simulink model "cost_function_only"  (R2022a)
settings: Solver=FixedStepDiscrete  StartTime=0.0  StopTime=10.0  RelTol=1e-3
undefined symbols (not defined in the file or in its folder): f_c
libraries: hdlsllib x1
settings Model: DataTypeOverride=Off  Creator=Andre Merx  LastModifiedBy=Andre Merx
settings SolverCC: AlgebraicLoopSolver=TrustRegion
settings DataIOCC: LimitDataPoints=on  SaveOutput=off  SaveTime=off
settings OptimizationCC: BlockReduction=off  ConditionallyExecuteInputs=off  DefaultParameterBehavior=Inlined  LifeSpan=inf
settings DebuggingCC: AlgebraicLoopMsg=error  SingleTaskRateTransMsg=error  UnconnectedInputMsg=warning  UnconnectedOutputMsg=warning  UnconnectedLineMsg=warning  AllowSymbolicDim=off  StrictBusMsg=ErrorOnBusTreatedAsVector  SFUnexpectedBacktrackingDiag=warning  SFNoUnconditionalDefaultTransitionDiag=warning  SFExecutionAtInitializationDiag=none  SFMachineParentedDataDiag=warning  ArithmeticOperatorsInVariantConditions=warning
settings HardwareCC: ProdBitPerPointer=32  ProdBitPerSizeT=32  ProdBitPerPtrDiffT=32  ProdLargestAtomicFloat=None  ProdIntDivRoundTo=Undefined  ProdEndianess=Unspecified  ProdWordSize=32  ProdHWDeviceType=ASIC/FPGA->ASIC/FPGA  ProdEqTarget=off
settings SFSimCC: SimUseLocalCustomCode=off  CustomCodeUndefinedFunction=UseInterfaceOnly
settings RTWCC: RTWUseLocalCustomCode=off
settings CodeAppCC: StateflowObjectComments=on
settings GRTTargetCC: TargetLangStandard=C89/C90 (ANSI)
settings ConfigComp: CovScope=ReferencedModels  CovMetricSettings=dw  CovSaveCumulativeToWorkspaceVar=on  CovSaveSingleToWorkspaceVar=on  CovExternalEMLEnable=off  CovSFcnEnable=off

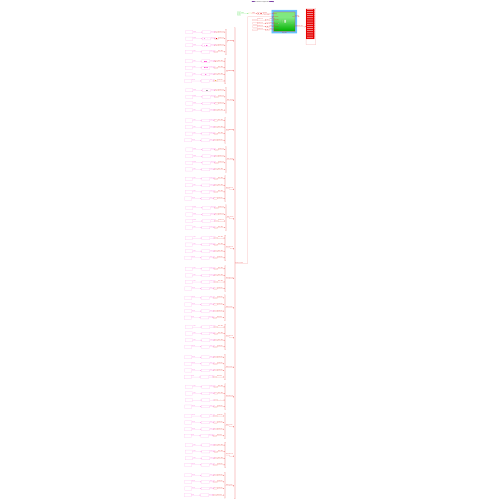
[thumbnail: Simulink's stored preview of the top-level diagram]
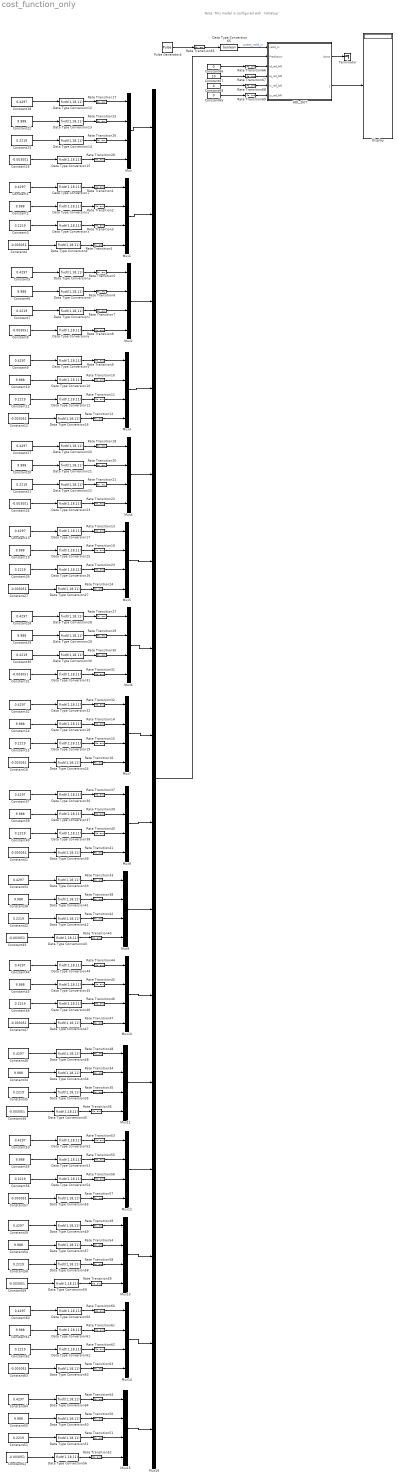
== system cost_function_only ==
  note: Note: This model is configured with ' hdlsetup '
  Constant{1,5,9,13,17..18,28,32..33,37,44,48..49,53,60,64} (16 alike) : Constant  Value=0.4297
  Constant{2,6,10,14,19..20,22,29,34,38..39,45,50,54..55,61} (16 alike) : Constant  Value=9.988
  Constant{3,7,11,15,21,23,26,30,35,40,42,46,51,56,58,62} (16 alike) : Constant  Value=0.2219
  Constant{4,8,12,16,24..25,27,31,36,41,43,47,52,57,59,63} (16 alike) : Constant  Value=-0.003051
  Constant65 : Constant  Value=0  OutDataTypeStr=fixdt(1,18,11)  SampleTime=-1
  Constant66 : Constant  Value=0  OutDataTypeStr=fixdt(1,18,11)  SampleTime=-1
  Constant67 : Constant  Value=10  OutDataTypeStr=fixdt(1,18,11)  SampleTime=-1
  Constant68 : Constant  Value=0  OutDataTypeStr=fixdt(1,18,11)  SampleTime=-1
  Data Type Conversion{1..64} (64 alike) : DataTypeConversion  OutDataTypeStr=fixdt(1,18,11)  SaturateOnIntegerOverflow=off  RndMeth=Floor
  Data Type Conversion65 : DataTypeConversion  OutDataTypeStr=boolean  SaturateOnIntegerOverflow=off  RndMeth=Floor
  Display : Display
  HDL_DUT : Subsystem  TreatAsAtomicUnit=on
  Mux{,1..15} (16 alike) : Mux
  Mux16 : Mux  Inputs=16
  Pulse Generator4 : DiscretePulseGenerator  PulseType=Time based  Period=1/f_c
  Rate Transition{1..69} (69 alike) : RateTransition  OutPortSampleTime=Rt
  Terminator : Terminator
  wires:
  Rate Transition17/1 -> Mux/1
  Constant25/1 -> Data Type Conversion15/1
  Rate Transition26/1 -> Mux/3
  Data Type Conversion12/1 -> Rate Transition17/1
  Rate Transition28/1 -> Mux/4
  Data Type Conversion13/1 -> Rate Transition25/1
  Data Type Conversion15/1 -> Rate Transition28/1
  Rate Transition25/1 -> Mux/2
  Constant18/1 -> Data Type Conversion12/1
  Constant23/1 -> Data Type Conversion14/1
  Constant22/1 -> Data Type Conversion13/1
  Data Type Conversion14/1 -> Rate Transition26/1
  Rate Transition4/1 -> Mux1/4
  Rate Transition3/1 -> Mux1/3
  Rate Transition2/1 -> Mux1/2
  Rate Transition1/1 -> Mux1/1
  Constant2/1 -> Data Type Conversion2/1
  Constant1/1 -> Data Type Conversion1/1
  Data Type Conversion4/1 -> Rate Transition4/1
  Constant3/1 -> Data Type Conversion3/1
  Data Type Conversion2/1 -> Rate Transition2/1
  Data Type Conversion1/1 -> Rate Transition1/1
  Constant4/1 -> Data Type Conversion4/1
  Data Type Conversion3/1 -> Rate Transition3/1
  Rate Transition8/1 -> Mux2/4
  Rate Transition7/1 -> Mux2/3
  Rate Transition6/1 -> Mux2/2
  Rate Transition5/1 -> Mux2/1
  Constant6/1 -> Data Type Conversion6/1
  Constant5/1 -> Data Type Conversion5/1
  Data Type Conversion8/1 -> Rate Transition8/1
  Constant7/1 -> Data Type Conversion7/1
  Data Type Conversion6/1 -> Rate Transition6/1
  Data Type Conversion5/1 -> Rate Transition5/1
  Constant8/1 -> Data Type Conversion8/1
  Data Type Conversion7/1 -> Rate Transition7/1
  Rate Transition12/1 -> Mux3/4
  Rate Transition11/1 -> Mux3/3
  Rate Transition10/1 -> Mux3/2
  Rate Transition9/1 -> Mux3/1
  Constant10/1 -> Data Type Conversion10/1
  Constant9/1 -> Data Type Conversion9/1
  Data Type Conversion16/1 -> Rate Transition12/1
  Constant11/1 -> Data Type Conversion11/1
  Data Type Conversion10/1 -> Rate Transition10/1
  Data Type Conversion9/1 -> Rate Transition9/1
  Constant12/1 -> Data Type Conversion16/1
  Data Type Conversion11/1 -> Rate Transition11/1
  Rate Transition22/1 -> Mux4/4
  Rate Transition21/1 -> Mux4/3
  Rate Transition20/1 -> Mux4/2
  Data Type Conversion20/1 -> Rate Transition18/1
  Constant17/1 -> Data Type Conversion20/1
  Constant21/1 -> Data Type Conversion22/1
  Data Type Conversion21/1 -> Rate Transition20/1
  Data Type Conversion22/1 -> Rate Transition21/1
  Data Type Conversion30/1 -> Rate Transition30/1
  Constant31/1 -> Data Type Conversion31/1
  Constant24/1 -> Data Type Conversion23/1
  Data Type Conversion28/1 -> Rate Transition27/1
  Data Type Conversion29/1 -> Rate Transition29/1
  Constant30/1 -> Data Type Conversion30/1
  Constant20/1 -> Data Type Conversion21/1
  Constant28/1 -> Data Type Conversion28/1
  Data Type Conversion31/1 -> Rate Transition31/1
  Rate Transition27/1 -> Mux6/1
  Rate Transition29/1 -> Mux6/2
  Rate Transition30/1 -> Mux6/3
  Rate Transition31/1 -> Mux6/4
  Rate Transition24/1 -> Mux5/4
  Data Type Conversion17/1 -> Rate Transition13/1
  Data Type Conversion25/1 -> Rate Transition19/1
  Constant19/1 -> Data Type Conversion25/1
  Rate Transition13/1 -> Mux5/1
  Constant26/1 -> Data Type Conversion26/1
  Rate Transition19/1 -> Mux5/2
  Rate Transition23/1 -> Mux5/3
  Rate Transition18/1 -> Mux4/1
  Constant16/1 -> Data Type Conversion24/1
  Data Type Conversion19/1 -> Rate Transition15/1
  Data Type Conversion23/1 -> Rate Transition22/1
  Data Type Conversion18/1 -> Rate Transition14/1
  Data Type Conversion26/1 -> Rate Transition23/1
  Data Type Conversion32/1 -> Rate Transition32/1
  Constant13/1 -> Data Type Conversion17/1
  Data Type Conversion24/1 -> Rate Transition16/1
  Constant32/1 -> Data Type Conversion32/1
  Constant14/1 -> Data Type Conversion18/1
  Constant15/1 -> Data Type Conversion19/1
  Constant29/1 -> Data Type Conversion29/1
  Rate Transition15/1 -> Mux7/3
  Constant27/1 -> Data Type Conversion27/1
  Rate Transition14/1 -> Mux7/2
  Rate Transition16/1 -> Mux7/4
  Data Type Conversion27/1 -> Rate Transition24/1
  Rate Transition32/1 -> Mux7/1
  Rate Transition41/1 -> Mux8/4
  Rate Transition40/1 -> Mux8/3
  Rate Transition39/1 -> Mux8/2
  Data Type Conversion36/1 -> Rate Transition37/1
  Constant37/1 -> Data Type Conversion36/1
  Constant40/1 -> Data Type Conversion38/1
  Data Type Conversion37/1 -> Rate Transition39/1
  Data Type Conversion38/1 -> Rate Transition40/1
  Data Type Conversion46/1 -> Rate Transition46/1
  Constant47/1 -> Data Type Conversion47/1
  Constant41/1 -> Data Type Conversion39/1
  Data Type Conversion44/1 -> Rate Transition44/1
  Data Type Conversion45/1 -> Rate Transition45/1
  Constant46/1 -> Data Type Conversion46/1
  Constant39/1 -> Data Type Conversion37/1
  Constant44/1 -> Data Type Conversion44/1
  Data Type Conversion47/1 -> Rate Transition47/1
  Rate Transition44/1 -> Mux10/1
  Rate Transition45/1 -> Mux10/2
  Rate Transition46/1 -> Mux10/3
  Rate Transition47/1 -> Mux10/4
  Rate Transition43/1 -> Mux9/4
  Data Type Conversion33/1 -> Rate Transition33/1
  Data Type Conversion41/1 -> Rate Transition38/1
  Constant38/1 -> Data Type Conversion41/1
  Rate Transition33/1 -> Mux9/1
  Constant42/1 -> Data Type Conversion42/1
  Rate Transition38/1 -> Mux9/2
  Rate Transition42/1 -> Mux9/3
  Rate Transition37/1 -> Mux8/1
  Constant36/1 -> Data Type Conversion40/1
  Data Type Conversion35/1 -> Rate Transition35/1
  Data Type Conversion39/1 -> Rate Transition41/1
  Data Type Conversion34/1 -> Rate Transition34/1
  Data Type Conversion42/1 -> Rate Transition42/1
  Data Type Conversion48/1 -> Rate Transition48/1
  Constant33/1 -> Data Type Conversion33/1
  Data Type Conversion40/1 -> Rate Transition36/1
  Constant48/1 -> Data Type Conversion48/1
  Constant34/1 -> Data Type Conversion34/1
  Constant35/1 -> Data Type Conversion35/1
  Constant45/1 -> Data Type Conversion45/1
  Rate Transition35/1 -> Mux11/3
  Constant43/1 -> Data Type Conversion43/1
  Rate Transition34/1 -> Mux11/2
  Rate Transition36/1 -> Mux11/4
  Data Type Conversion43/1 -> Rate Transition43/1
  Rate Transition48/1 -> Mux11/1
  Rate Transition57/1 -> Mux12/4
  Rate Transition56/1 -> Mux12/3
  Rate Transition55/1 -> Mux12/2
  Data Type Conversion52/1 -> Rate Transition53/1
  Constant53/1 -> Data Type Conversion52/1
  Constant56/1 -> Data Type Conversion54/1
  Data Type Conversion53/1 -> Rate Transition55/1
  Data Type Conversion54/1 -> Rate Transition56/1
  Data Type Conversion62/1 -> Rate Transition62/1
  Constant63/1 -> Data Type Conversion63/1
  Constant57/1 -> Data Type Conversion55/1
  Data Type Conversion60/1 -> Rate Transition60/1
  Data Type Conversion61/1 -> Rate Transition61/1
  Constant62/1 -> Data Type Conversion62/1
  Constant55/1 -> Data Type Conversion53/1
  Constant60/1 -> Data Type Conversion60/1
  Data Type Conversion63/1 -> Rate Transition63/1
  Rate Transition60/1 -> Mux14/1
  Rate Transition61/1 -> Mux14/2
  Rate Transition62/1 -> Mux14/3
  Rate Transition63/1 -> Mux14/4
  Rate Transition59/1 -> Mux13/4
  Data Type Conversion49/1 -> Rate Transition49/1
  Data Type Conversion57/1 -> Rate Transition54/1
  Constant54/1 -> Data Type Conversion57/1
  Rate Transition49/1 -> Mux13/1
  Constant58/1 -> Data Type Conversion58/1
  Rate Transition54/1 -> Mux13/2
  Rate Transition58/1 -> Mux13/3
  Rate Transition53/1 -> Mux12/1
  Constant52/1 -> Data Type Conversion56/1
  Data Type Conversion51/1 -> Rate Transition51/1
  Data Type Conversion55/1 -> Rate Transition57/1
  Data Type Conversion50/1 -> Rate Transition50/1
  Data Type Conversion58/1 -> Rate Transition58/1
  Data Type Conversion64/1 -> Rate Transition64/1
  Constant49/1 -> Data Type Conversion49/1
  Data Type Conversion56/1 -> Rate Transition52/1
  Constant64/1 -> Data Type Conversion64/1
  Constant50/1 -> Data Type Conversion50/1
  Constant51/1 -> Data Type Conversion51/1
  Constant61/1 -> Data Type Conversion61/1
  Rate Transition51/1 -> Mux15/3
  Constant59/1 -> Data Type Conversion59/1
  Rate Transition50/1 -> Mux15/2
  Rate Transition52/1 -> Mux15/4
  Data Type Conversion59/1 -> Rate Transition59/1
  Rate Transition64/1 -> Mux15/1
  Mux/1 -> Mux16/1
  Mux1/1 -> Mux16/2
  Mux2/1 -> Mux16/3
  Mux3/1 -> Mux16/4
  Mux4/1 -> Mux16/5
  Mux5/1 -> Mux16/6
  Mux6/1 -> Mux16/7
  Mux7/1 -> Mux16/8
  Mux8/1 -> Mux16/9
  Mux9/1 -> Mux16/10
  Mux10/1 -> Mux16/11
  Mux11/1 -> Mux16/12
  Mux12/1 -> Mux16/13
  Mux13/1 -> Mux16/14
  Mux14/1 -> Mux16/15
  Mux15/1 -> Mux16/16
  Mux16/1 -> HDL_DUT/2(Prediction)
  Data Type Conversion65/1 -> HDL_DUT/1(valid_in)  "curent_valid_in"
  Pulse Generator4/1 -> Rate Transition65/1
  Rate Transition65/1 -> Data Type Conversion65/1
  Constant67/1 -> Rate Transition67/1
  Constant66/1 -> Rate Transition66/1
  Rate Transition66/1 -> HDL_DUT/3(id_ref_AXI)
  Constant68/1 -> Rate Transition68/1
  Rate Transition68/1 -> HDL_DUT/5(ix_ref_AXI)
  Rate Transition67/1 -> HDL_DUT/4(iq_ref_AXI)
  Rate Transition69/1 -> HDL_DUT/6(iy_ref_AXI)
  Constant65/1 -> Rate Transition69/1
  HDL_DUT/1(done) -> Terminator/1
  HDL_DUT/2(J) -> Display/1

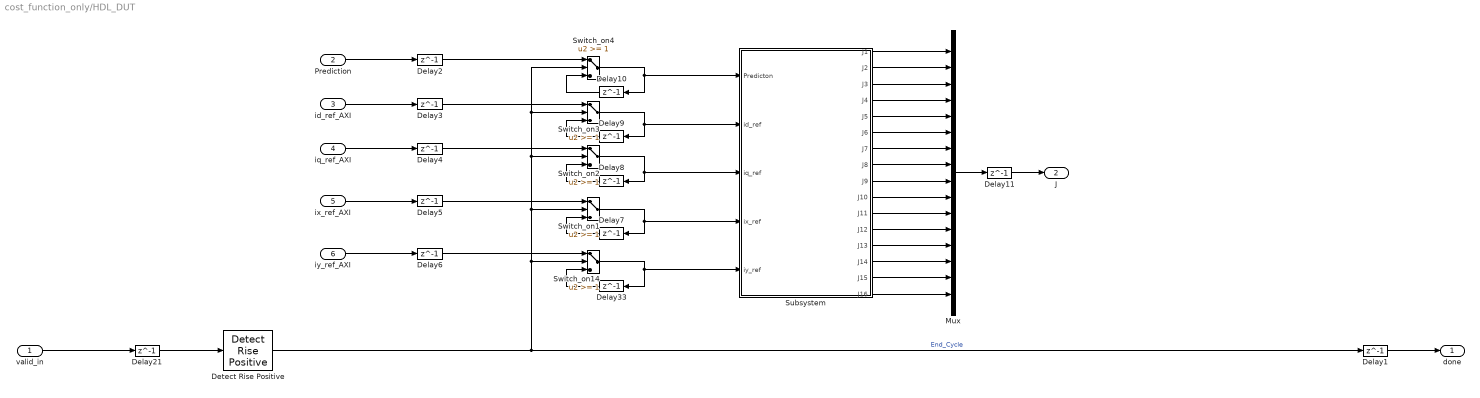
== system cost_function_only/HDL_DUT ==
  valid_in : Inport
  Prediction : Inport  Port=2
  id_ref_AXI : Inport  Port=3
  iq_ref_AXI : Inport  Port=4
  ix_ref_AXI : Inport  Port=5
  iy_ref_AXI : Inport  Port=6
  Delay{1..11,21,33} (13 alike) : Delay  DelayLength=1
  Detect Rise Positive : hdlsllib/Logic and Bit Operations/Detect Rise Positive  vinit=0  OutDataTypeStr=boolean
      settings: SourceProductBaseCode=SL
  Mux : Mux  Inputs=16
  Subsystem : Subsystem
  Switch_on{1..4,14} (5 alike) : Switch  Threshold=1  OutDataTypeStr=fixdt(1,18,11)  RndMeth=Simplest  SaturateOnIntegerOverflow=off  InputSameDT=off
  done : Outport
  J : Outport  Port=2
  wires:
  Delay21/1 -> Detect Rise Positive/1
  valid_in/1 -> Delay21/1
  Delay1/1 -> done/1
  Prediction/1 -> Delay2/1
  id_ref_AXI/1 -> Delay3/1
  iq_ref_AXI/1 -> Delay4/1
  ix_ref_AXI/1 -> Delay5/1
  iy_ref_AXI/1 -> Delay6/1
  Delay6/1 -> Switch_on14/1
  Switch_on14/1 -> Delay33/1, Subsystem/5(iy_ref)
  Delay33/1 -> Switch_on14/3
  Delay7/1 -> Switch_on1/3
  Delay5/1 -> Switch_on1/1
  Switch_on1/1 -> Subsystem/4(ix_ref), Delay7/1
  Delay8/1 -> Switch_on2/3
  Delay4/1 -> Switch_on2/1
  Switch_on2/1 -> Subsystem/3(iq_ref), Delay8/1
  Delay9/1 -> Switch_on3/3
  Delay3/1 -> Switch_on3/1
  Switch_on3/1 -> Subsystem/2(id_ref), Delay9/1
  Delay10/1 -> Switch_on4/3
  Detect Rise Positive/1 -> Switch_on4/2, Switch_on3/2, Switch_on2/2, Switch_on1/2, Switch_on14/2, Delay1/1  "End_Cycle"
  Delay2/1 -> Switch_on4/1
  Switch_on4/1 -> Delay10/1, Subsystem/1(Predicton)
  Subsystem/1(J1) -> Mux/1
  Subsystem/2(J2) -> Mux/2
  Subsystem/3(J3) -> Mux/3
  Subsystem/4(J4) -> Mux/4
  Subsystem/5(J5) -> Mux/5
  Subsystem/6(J6) -> Mux/6
  Subsystem/7(J7) -> Mux/7
  Subsystem/8(J8) -> Mux/8
  Subsystem/9(J9) -> Mux/9
  Subsystem/10(J10) -> Mux/10
  Subsystem/11(J11) -> Mux/11
  Subsystem/12(J12) -> Mux/12
  Subsystem/13(J13) -> Mux/13
  Subsystem/14(J14) -> Mux/14
  Subsystem/15(J15) -> Mux/15
  Subsystem/16(J16) -> Mux/16
  Mux/1 -> Delay11/1
  Delay11/1 -> J/1

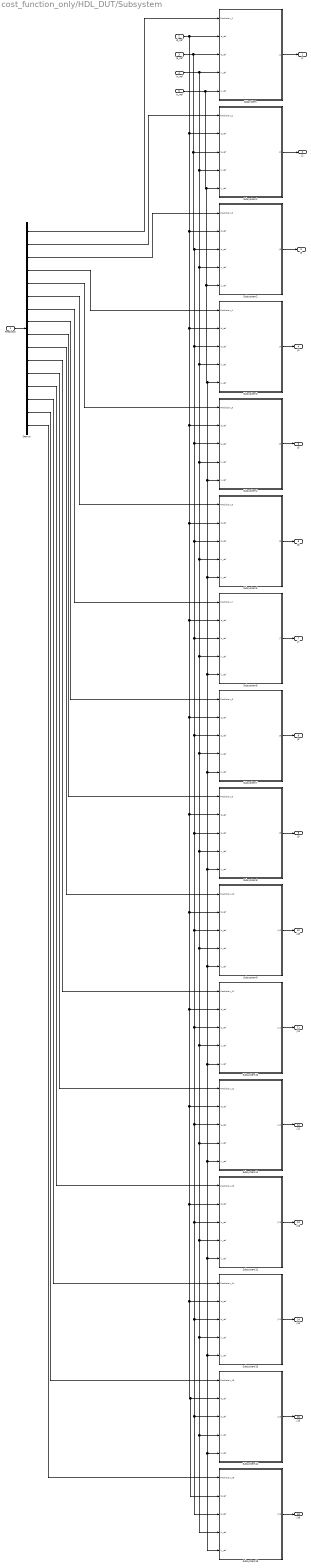
== system cost_function_only/HDL_DUT/Subsystem ==
  Predicton : Inport
  id_ref : Inport  Port=2
  iq_ref : Inport  Port=3
  ix_ref : Inport  Port=4
  iy_ref : Inport  Port=5
  Demux : Demux  Outputs=16
  Subsystem : Subsystem
  Subsystem1 : Subsystem
  Subsystem10 : Subsystem
  Subsystem11 : Subsystem
  Subsystem12 : Subsystem
  Subsystem13 : Subsystem
  Subsystem14 : Subsystem
  Subsystem15 : Subsystem
  Subsystem2 : Subsystem
  Subsystem3 : Subsystem
  Subsystem4 : Subsystem
  Subsystem5 : Subsystem
  Subsystem6 : Subsystem
  Subsystem7 : Subsystem
  Subsystem8 : Subsystem
  Subsystem9 : Subsystem
  J1 : Outport
  J2 : Outport  Port=2
  J3 : Outport  Port=3
  J4 : Outport  Port=4
  J5 : Outport  Port=5
  J6 : Outport  Port=6
  J7 : Outport  Port=7
  J8 : Outport  Port=8
  J9 : Outport  Port=9
  J10 : Outport  Port=10
  J11 : Outport  Port=11
  J12 : Outport  Port=12
  J13 : Outport  Port=13
  J14 : Outport  Port=14
  J15 : Outport  Port=15
  J16 : Outport  Port=16
  wires:
  Predicton/1 -> Demux/1
  iy_ref/1 -> Subsystem/5(iy_ref), Subsystem15/5(iy_ref), Subsystem14/5(iy_ref), Subsystem13/5(iy_ref), Subsystem12/5(iy_ref), Subsystem11/5(iy_ref), Subsystem10/5(iy_ref), Subsystem9/5(iy_ref), Subsystem8/5(iy_ref), Subsystem7/5(iy_ref), Subsystem6/5(iy_ref), Subsystem5/5(iy_ref), Subsystem4/5(iy_ref), Subsystem3/5(iy_ref), Subsystem2/5(iy_ref), Subsystem1/5(iy_ref)
  ix_ref/1 -> Subsystem/4(ix_ref), Subsystem15/4(ix_ref), Subsystem14/4(ix_ref), Subsystem13/4(ix_ref), Subsystem12/4(ix_ref), Subsystem11/4(ix_ref), Subsystem10/4(ix_ref), Subsystem9/4(ix_ref), Subsystem8/4(ix_ref), Subsystem7/4(ix_ref), Subsystem6/4(ix_ref), Subsystem5/4(ix_ref), Subsystem4/4(ix_ref), Subsystem3/4(ix_ref), Subsystem2/4(ix_ref), Subsystem1/4(ix_ref)
  iq_ref/1 -> Subsystem/3(iq_ref), Subsystem15/3(iq_ref), Subsystem14/3(iq_ref), Subsystem13/3(iq_ref), Subsystem12/3(iq_ref), Subsystem11/3(iq_ref), Subsystem10/3(iq_ref), Subsystem9/3(iq_ref), Subsystem8/3(iq_ref), Subsystem7/3(iq_ref), Subsystem6/3(iq_ref), Subsystem5/3(iq_ref), Subsystem4/3(iq_ref), Subsystem3/3(iq_ref), Subsystem2/3(iq_ref), Subsystem1/3(iq_ref)
  id_ref/1 -> Subsystem15/2(id_ref), Subsystem14/2(id_ref), Subsystem13/2(id_ref), Subsystem12/2(id_ref), Subsystem11/2(id_ref), Subsystem10/2(id_ref), Subsystem9/2(id_ref), Subsystem8/2(id_ref), Subsystem7/2(id_ref), Subsystem6/2(id_ref), Subsystem5/2(id_ref), Subsystem4/2(id_ref), Subsystem3/2(id_ref), Subsystem2/2(id_ref), Subsystem1/2(id_ref), Subsystem/2(id_ref)
  Demux/1 -> Subsystem/1(Prediction_1)
  Demux/2 -> Subsystem1/1(Prediction_2)
  Demux/3 -> Subsystem2/1(Prediction_3)
  Demux/4 -> Subsystem3/1(Prediction_4)
  Demux/5 -> Subsystem4/1(Prediction_5)
  Demux/6 -> Subsystem5/1(Prediction_6)
  Demux/7 -> Subsystem6/1(Prediction_7)
  Demux/8 -> Subsystem7/1(Prediction_8)
  Demux/9 -> Subsystem8/1(Prediction_9)
  Demux/10 -> Subsystem9/1(Prediction_10)
  Demux/11 -> Subsystem10/1(Prediction_11)
  Demux/12 -> Subsystem11/1(Prediction_12)
  Demux/13 -> Subsystem12/1(Prediction_13)
  Demux/14 -> Subsystem13/1(Prediction_14)
  Demux/15 -> Subsystem14/1(Prediction_15)
  Demux/16 -> Subsystem15/1(Prediction_16)
  Subsystem/1(J1) -> J1/1
  Subsystem1/1(J2) -> J2/1
  Subsystem2/1(J3) -> J3/1
  Subsystem3/1(J4) -> J4/1
  Subsystem4/1(J5) -> J5/1
  Subsystem5/1(J6) -> J6/1
  Subsystem6/1(J7) -> J7/1
  Subsystem7/1(J8) -> J8/1
  Subsystem8/1(J9) -> J9/1
  Subsystem9/1(J10) -> J10/1
  Subsystem10/1(J11) -> J11/1
  Subsystem11/1(J12) -> J12/1
  Subsystem12/1(J13) -> J13/1
  Subsystem13/1(J14) -> J14/1
  Subsystem14/1(J15) -> J15/1
  Subsystem15/1(J16) -> J16/1

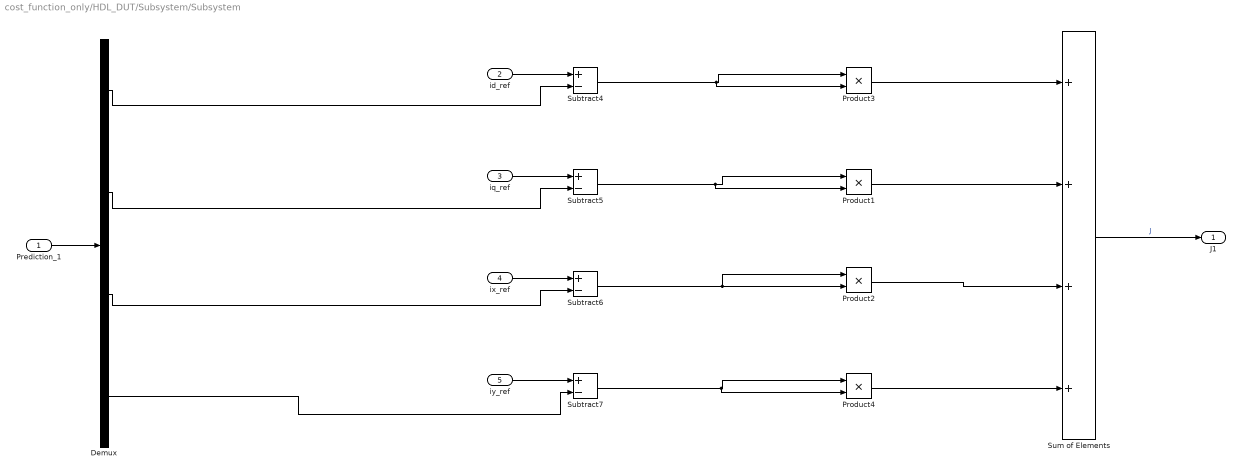
== system cost_function_only/HDL_DUT/Subsystem/Subsystem ==
  Prediction_1 : Inport
  id_ref : Inport  Port=2
  iq_ref : Inport  Port=3
  ix_ref : Inport  Port=4
  iy_ref : Inport  Port=5
  Demux : Demux
  Product{1..4} (4 alike) : Product  OutDataTypeStr=fixdt(1,20,11)
  Subtract{4..7} (4 alike) : Sum  Inputs=+-  OutDataTypeStr=fixdt(1,20,11)
  Sum of Elements : Sum  Inputs=++++  OutDataTypeStr=fixdt(1,20,11)
  J1 : Outport
  wires:
  Prediction_1/1 -> Demux/1
  iy_ref/1 -> Subtract7/1
  Demux/3 -> Subtract6/2
  Sum of Elements/1 -> J1/1  "J"
  iq_ref/1 -> Subtract5/1
  id_ref/1 -> Subtract4/1
  Demux/2 -> Subtract5/2
  ix_ref/1 -> Subtract6/1
  Demux/4 -> Subtract7/2
  Demux/1 -> Subtract4/2
  Product3/1 -> Sum of Elements/1
  Product1/1 -> Sum of Elements/2
  Product2/1 -> Sum of Elements/3
  Product4/1 -> Sum of Elements/4
  Subtract4/1 -> Product3/2, Product3/1
  Subtract5/1 -> Product1/2, Product1/1
  Subtract6/1 -> Product2/2, Product2/1
  Subtract7/1 -> Product4/2, Product4/1

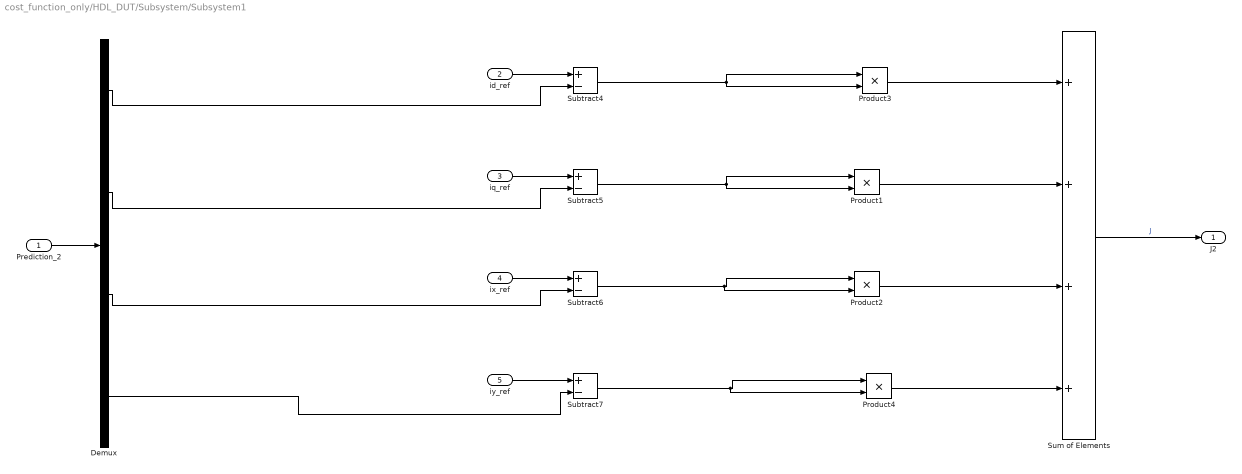
== system cost_function_only/HDL_DUT/Subsystem/Subsystem1 ==
  Prediction_2 : Inport
  id_ref : Inport  Port=2
  iq_ref : Inport  Port=3
  ix_ref : Inport  Port=4
  iy_ref : Inport  Port=5
  Demux : Demux
  Product{1..4} (4 alike) : Product  OutDataTypeStr=fixdt(1,20,11)
  Subtract{4..7} (4 alike) : Sum  Inputs=+-  OutDataTypeStr=fixdt(1,20,11)
  Sum of Elements : Sum  Inputs=++++  OutDataTypeStr=fixdt(1,20,11)
  J2 : Outport
  wires:
  Prediction_2/1 -> Demux/1
  iy_ref/1 -> Subtract7/1
  Demux/3 -> Subtract6/2
  Sum of Elements/1 -> J2/1  "J"
  iq_ref/1 -> Subtract5/1
  id_ref/1 -> Subtract4/1
  Demux/2 -> Subtract5/2
  ix_ref/1 -> Subtract6/1
  Demux/4 -> Subtract7/2
  Demux/1 -> Subtract4/2
  Product3/1 -> Sum of Elements/1
  Product1/1 -> Sum of Elements/2
  Product2/1 -> Sum of Elements/3
  Product4/1 -> Sum of Elements/4
  Subtract4/1 -> Product3/2, Product3/1
  Subtract5/1 -> Product1/2, Product1/1
  Subtract6/1 -> Product2/2, Product2/1
  Subtract7/1 -> Product4/2, Product4/1

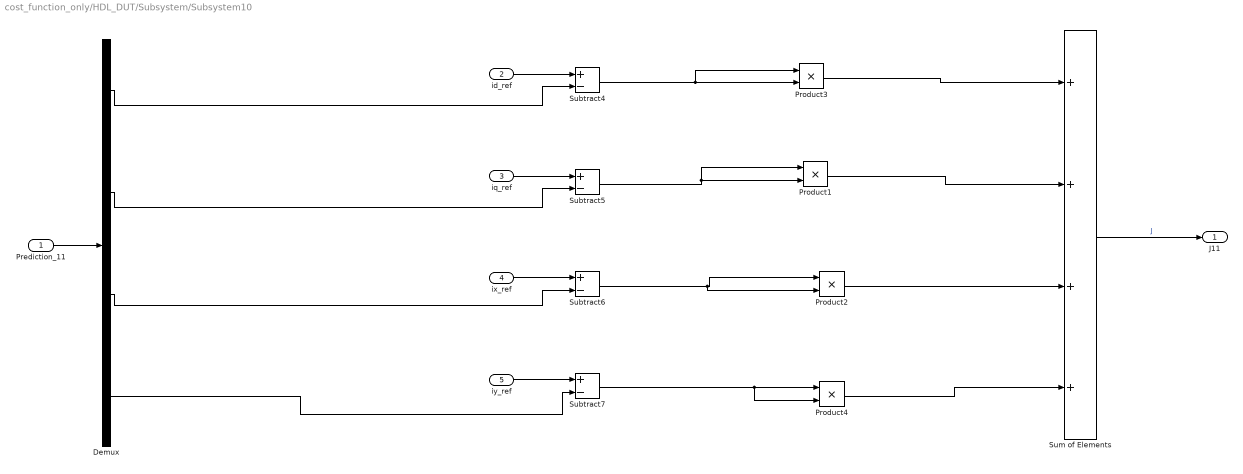
== system cost_function_only/HDL_DUT/Subsystem/Subsystem10 ==
  Prediction_11 : Inport
  id_ref : Inport  Port=2
  iq_ref : Inport  Port=3
  ix_ref : Inport  Port=4
  iy_ref : Inport  Port=5
  Demux : Demux
  Product{1..4} (4 alike) : Product  OutDataTypeStr=fixdt(1,20,11)
  Subtract{4..7} (4 alike) : Sum  Inputs=+-  OutDataTypeStr=fixdt(1,20,11)
  Sum of Elements : Sum  Inputs=++++  OutDataTypeStr=fixdt(1,20,11)
  J11 : Outport
  wires:
  Prediction_11/1 -> Demux/1
  iy_ref/1 -> Subtract7/1
  Demux/3 -> Subtract6/2
  Sum of Elements/1 -> J11/1  "J"
  iq_ref/1 -> Subtract5/1
  id_ref/1 -> Subtract4/1
  Demux/2 -> Subtract5/2
  ix_ref/1 -> Subtract6/1
  Demux/4 -> Subtract7/2
  Demux/1 -> Subtract4/2
  Product3/1 -> Sum of Elements/1
  Product1/1 -> Sum of Elements/2
  Product2/1 -> Sum of Elements/3
  Product4/1 -> Sum of Elements/4
  Subtract4/1 -> Product3/2, Product3/1
  Subtract5/1 -> Product1/2, Product1/1
  Subtract6/1 -> Product2/2, Product2/1
  Subtract7/1 -> Product4/2, Product4/1

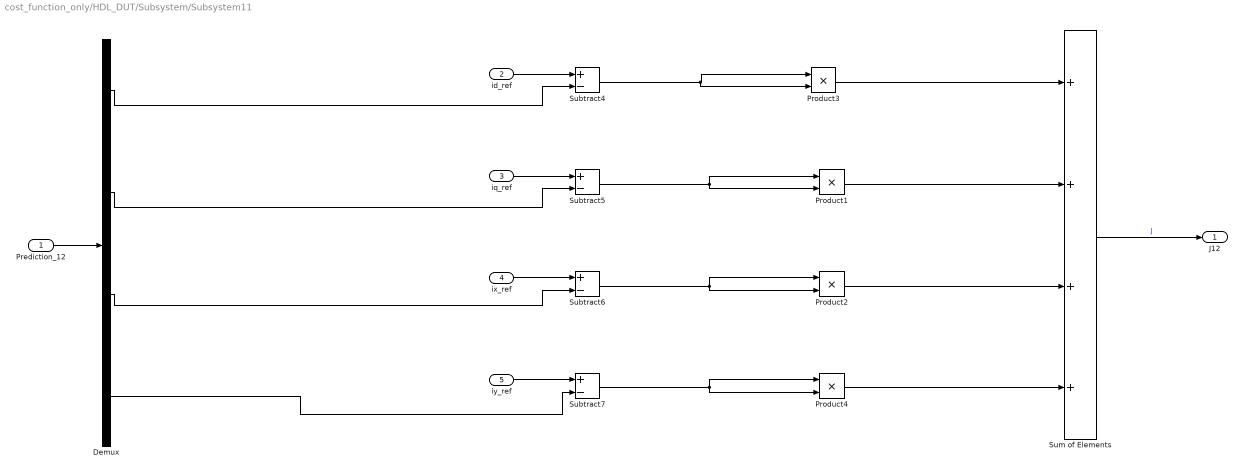
== system cost_function_only/HDL_DUT/Subsystem/Subsystem11 ==
  Prediction_12 : Inport
  id_ref : Inport  Port=2
  iq_ref : Inport  Port=3
  ix_ref : Inport  Port=4
  iy_ref : Inport  Port=5
  Demux : Demux
  Product{1..4} (4 alike) : Product  OutDataTypeStr=fixdt(1,20,11)
  Subtract{4..7} (4 alike) : Sum  Inputs=+-  OutDataTypeStr=fixdt(1,20,11)
  Sum of Elements : Sum  Inputs=++++  OutDataTypeStr=fixdt(1,20,11)
  J12 : Outport
  wires:
  Prediction_12/1 -> Demux/1
  iy_ref/1 -> Subtract7/1
  Demux/3 -> Subtract6/2
  Sum of Elements/1 -> J12/1  "J"
  iq_ref/1 -> Subtract5/1
  id_ref/1 -> Subtract4/1
  Demux/2 -> Subtract5/2
  ix_ref/1 -> Subtract6/1
  Demux/4 -> Subtract7/2
  Demux/1 -> Subtract4/2
  Product3/1 -> Sum of Elements/1
  Product1/1 -> Sum of Elements/2
  Product2/1 -> Sum of Elements/3
  Product4/1 -> Sum of Elements/4
  Subtract4/1 -> Product3/2, Product3/1
  Subtract5/1 -> Product1/1, Product1/2
  Subtract6/1 -> Product2/2, Product2/1
  Subtract7/1 -> Product4/2, Product4/1

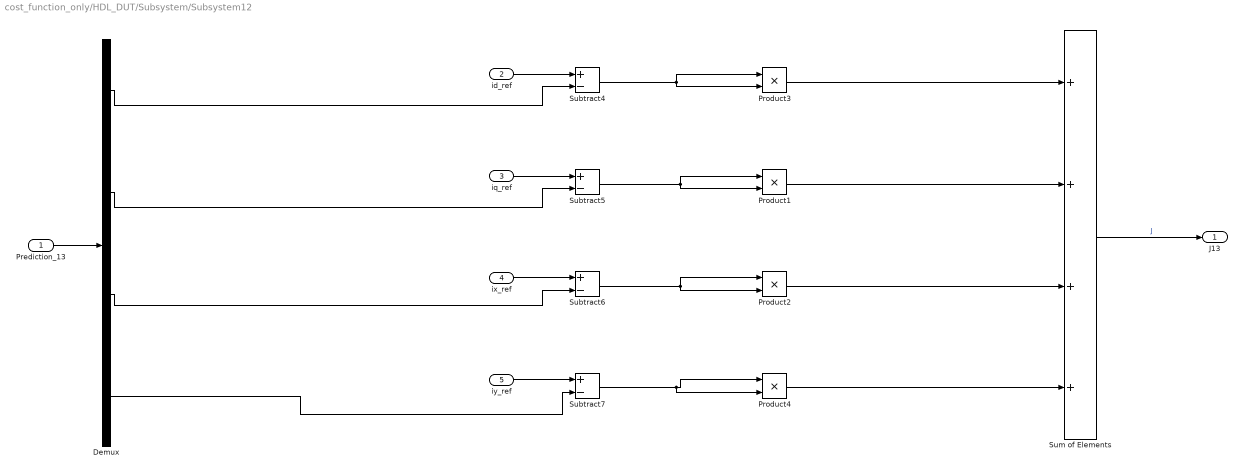
== system cost_function_only/HDL_DUT/Subsystem/Subsystem12 ==
  Prediction_13 : Inport
  id_ref : Inport  Port=2
  iq_ref : Inport  Port=3
  ix_ref : Inport  Port=4
  iy_ref : Inport  Port=5
  Demux : Demux
  Product{1..4} (4 alike) : Product  OutDataTypeStr=fixdt(1,20,11)
  Subtract{4..7} (4 alike) : Sum  Inputs=+-  OutDataTypeStr=fixdt(1,20,11)
  Sum of Elements : Sum  Inputs=++++  OutDataTypeStr=fixdt(1,20,11)
  J13 : Outport
  wires:
  Prediction_13/1 -> Demux/1
  iy_ref/1 -> Subtract7/1
  Demux/3 -> Subtract6/2
  Sum of Elements/1 -> J13/1  "J"
  iq_ref/1 -> Subtract5/1
  id_ref/1 -> Subtract4/1
  Demux/2 -> Subtract5/2
  ix_ref/1 -> Subtract6/1
  Demux/4 -> Subtract7/2
  Demux/1 -> Subtract4/2
  Product3/1 -> Sum of Elements/1
  Product1/1 -> Sum of Elements/2
  Product2/1 -> Sum of Elements/3
  Product4/1 -> Sum of Elements/4
  Subtract4/1 -> Product3/2, Product3/1
  Subtract5/1 -> Product1/2, Product1/1
  Subtract6/1 -> Product2/2, Product2/1
  Subtract7/1 -> Product4/2, Product4/1

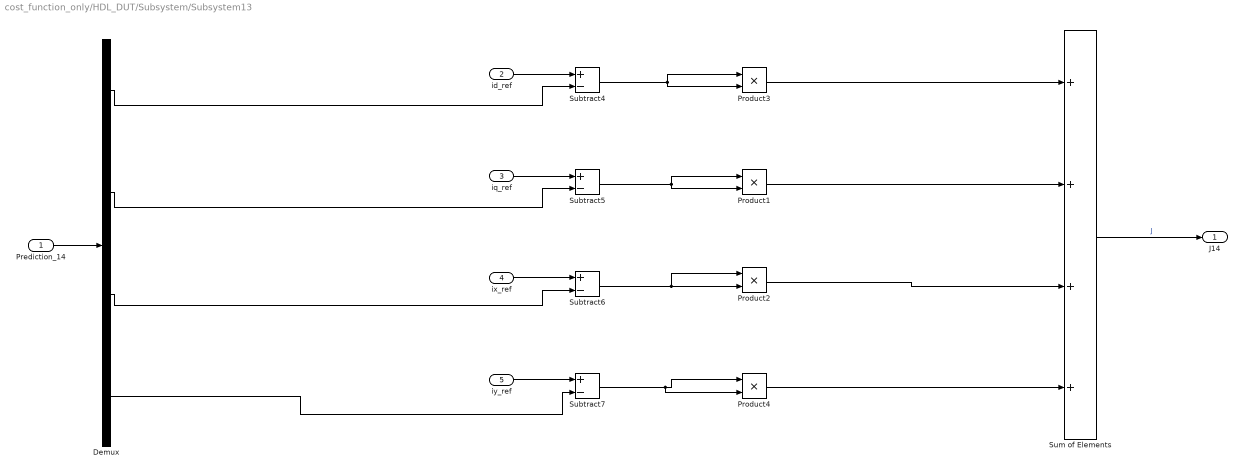
== system cost_function_only/HDL_DUT/Subsystem/Subsystem13 ==
  Prediction_14 : Inport
  id_ref : Inport  Port=2
  iq_ref : Inport  Port=3
  ix_ref : Inport  Port=4
  iy_ref : Inport  Port=5
  Demux : Demux
  Product{1..4} (4 alike) : Product  OutDataTypeStr=fixdt(1,20,11)
  Subtract{4..7} (4 alike) : Sum  Inputs=+-  OutDataTypeStr=fixdt(1,20,11)
  Sum of Elements : Sum  Inputs=++++  OutDataTypeStr=fixdt(1,20,11)
  J14 : Outport
  wires:
  Prediction_14/1 -> Demux/1
  iy_ref/1 -> Subtract7/1
  Demux/3 -> Subtract6/2
  Sum of Elements/1 -> J14/1  "J"
  iq_ref/1 -> Subtract5/1
  id_ref/1 -> Subtract4/1
  Demux/2 -> Subtract5/2
  ix_ref/1 -> Subtract6/1
  Demux/4 -> Subtract7/2
  Demux/1 -> Subtract4/2
  Product3/1 -> Sum of Elements/1
  Product1/1 -> Sum of Elements/2
  Product2/1 -> Sum of Elements/3
  Product4/1 -> Sum of Elements/4
  Subtract4/1 -> Product3/2, Product3/1
  Subtract5/1 -> Product1/1, Product1/2
  Subtract6/1 -> Product2/2, Product2/1
  Subtract7/1 -> Product4/2, Product4/1

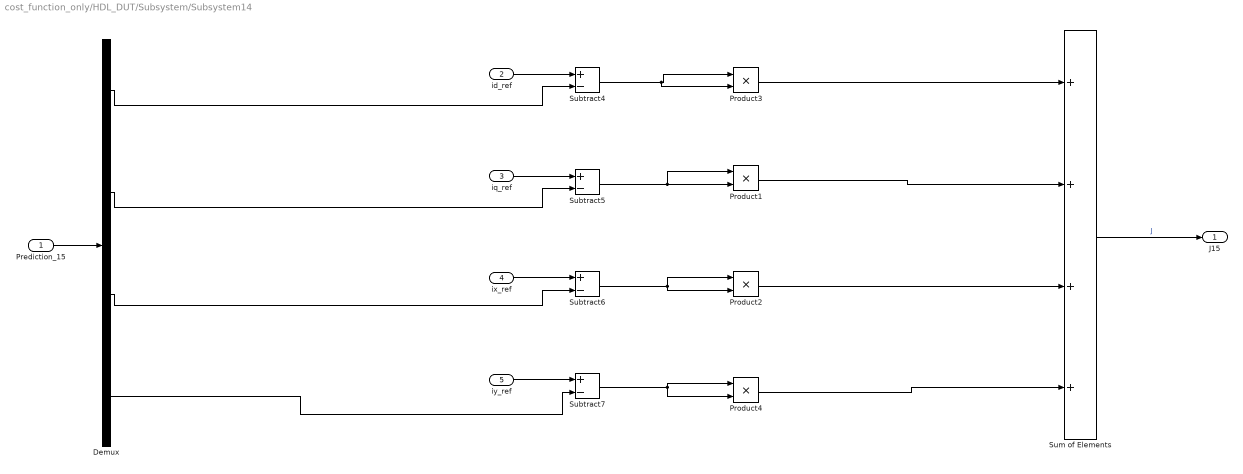
== system cost_function_only/HDL_DUT/Subsystem/Subsystem14 ==
  Prediction_15 : Inport
  id_ref : Inport  Port=2
  iq_ref : Inport  Port=3
  ix_ref : Inport  Port=4
  iy_ref : Inport  Port=5
  Demux : Demux
  Product{1..4} (4 alike) : Product  OutDataTypeStr=fixdt(1,20,11)
  Subtract{4..7} (4 alike) : Sum  Inputs=+-  OutDataTypeStr=fixdt(1,20,11)
  Sum of Elements : Sum  Inputs=++++  OutDataTypeStr=fixdt(1,20,11)
  J15 : Outport
  wires:
  Prediction_15/1 -> Demux/1
  iy_ref/1 -> Subtract7/1
  Demux/3 -> Subtract6/2
  Sum of Elements/1 -> J15/1  "J"
  iq_ref/1 -> Subtract5/1
  id_ref/1 -> Subtract4/1
  Demux/2 -> Subtract5/2
  ix_ref/1 -> Subtract6/1
  Demux/4 -> Subtract7/2
  Demux/1 -> Subtract4/2
  Product3/1 -> Sum of Elements/1
  Product1/1 -> Sum of Elements/2
  Product2/1 -> Sum of Elements/3
  Product4/1 -> Sum of Elements/4
  Subtract4/1 -> Product3/2, Product3/1
  Subtract5/1 -> Product1/1, Product1/2
  Subtract6/1 -> Product2/2, Product2/1
  Subtract7/1 -> Product4/2, Product4/1

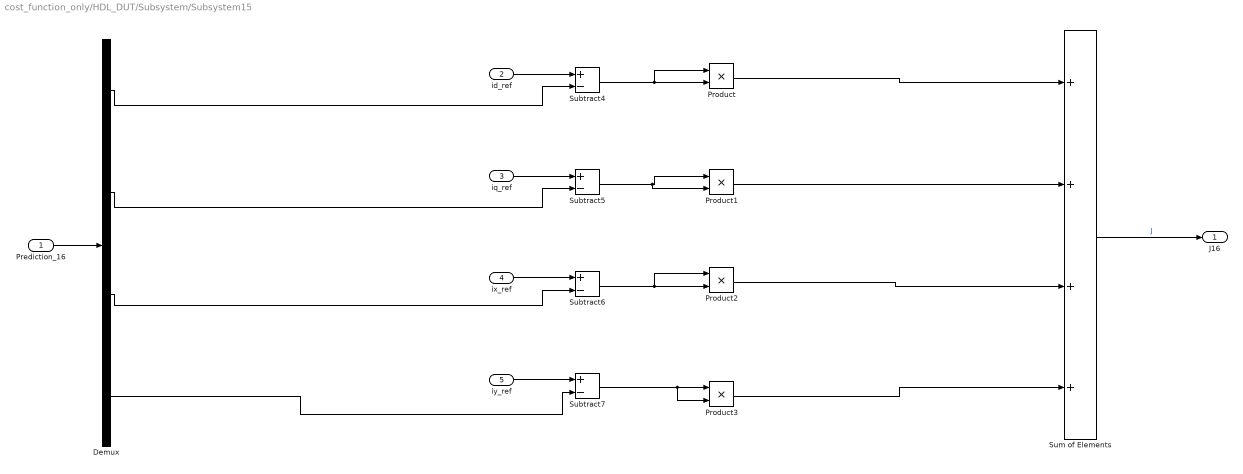
== system cost_function_only/HDL_DUT/Subsystem/Subsystem15 ==
  Prediction_16 : Inport
  id_ref : Inport  Port=2
  iq_ref : Inport  Port=3
  ix_ref : Inport  Port=4
  iy_ref : Inport  Port=5
  Demux : Demux
  Product{,1..3} (4 alike) : Product  OutDataTypeStr=fixdt(1,20,11)
  Subtract{4..7} (4 alike) : Sum  Inputs=+-  OutDataTypeStr=fixdt(1,20,11)
  Sum of Elements : Sum  Inputs=++++  OutDataTypeStr=fixdt(1,20,11)
  J16 : Outport
  wires:
  Prediction_16/1 -> Demux/1
  Product/1 -> Sum of Elements/1
  iy_ref/1 -> Subtract7/1
  Demux/3 -> Subtract6/2
  Sum of Elements/1 -> J16/1  "J"
  iq_ref/1 -> Subtract5/1
  id_ref/1 -> Subtract4/1
  Demux/2 -> Subtract5/2
  ix_ref/1 -> Subtract6/1
  Demux/4 -> Subtract7/2
  Demux/1 -> Subtract4/2
  Subtract4/1 -> Product/2, Product/1
  Subtract5/1 -> Product1/2, Product1/1
  Product1/1 -> Sum of Elements/2
  Product2/1 -> Sum of Elements/3
  Subtract6/1 -> Product2/1, Product2/2
  Subtract7/1 -> Product3/2, Product3/1
  Product3/1 -> Sum of Elements/4

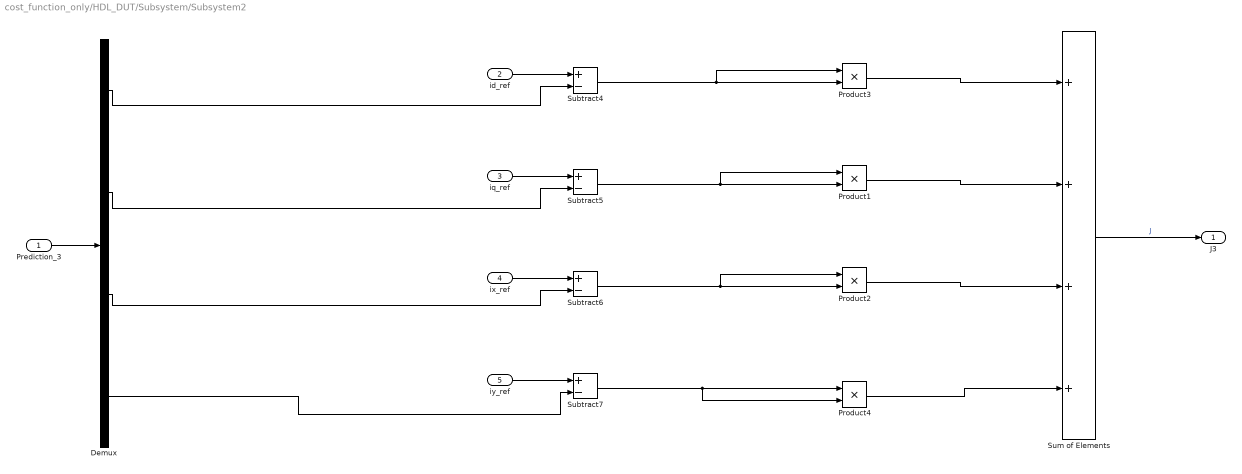
== system cost_function_only/HDL_DUT/Subsystem/Subsystem2 ==
  Prediction_3 : Inport
  id_ref : Inport  Port=2
  iq_ref : Inport  Port=3
  ix_ref : Inport  Port=4
  iy_ref : Inport  Port=5
  Demux : Demux
  Product{1..4} (4 alike) : Product  OutDataTypeStr=fixdt(1,20,11)
  Subtract{4..7} (4 alike) : Sum  Inputs=+-  OutDataTypeStr=fixdt(1,20,11)
  Sum of Elements : Sum  Inputs=++++  OutDataTypeStr=fixdt(1,20,11)
  J3 : Outport
  wires:
  Prediction_3/1 -> Demux/1
  iy_ref/1 -> Subtract7/1
  Demux/3 -> Subtract6/2
  Sum of Elements/1 -> J3/1  "J"
  iq_ref/1 -> Subtract5/1
  id_ref/1 -> Subtract4/1
  Demux/2 -> Subtract5/2
  ix_ref/1 -> Subtract6/1
  Demux/4 -> Subtract7/2
  Demux/1 -> Subtract4/2
  Product3/1 -> Sum of Elements/1
  Product1/1 -> Sum of Elements/2
  Product2/1 -> Sum of Elements/3
  Product4/1 -> Sum of Elements/4
  Subtract4/1 -> Product3/2, Product3/1
  Subtract5/1 -> Product1/2, Product1/1
  Subtract6/1 -> Product2/2, Product2/1
  Subtract7/1 -> Product4/2, Product4/1

== system cost_function_only/HDL_DUT/Subsystem/Subsystem3 ==
  Prediction_4 : Inport
  id_ref : Inport  Port=2
  iq_ref : Inport  Port=3
  ix_ref : Inport  Port=4
  iy_ref : Inport  Port=5
  Demux : Demux
  Product{1..4} (4 alike) : Product  OutDataTypeStr=fixdt(1,20,11)
  Subtract{4..7} (4 alike) : Sum  Inputs=+-  OutDataTypeStr=fixdt(1,20,11)
  Sum of Elements : Sum  Inputs=++++  OutDataTypeStr=fixdt(1,20,11)
  J4 : Outport
  wires:
  Prediction_4/1 -> Demux/1
  iy_ref/1 -> Subtract7/1
  Demux/3 -> Subtract6/2
  Sum of Elements/1 -> J4/1  "J"
  iq_ref/1 -> Subtract5/1
  id_ref/1 -> Subtract4/1
  Demux/2 -> Subtract5/2
  ix_ref/1 -> Subtract6/1
  Demux/4 -> Subtract7/2
  Demux/1 -> Subtract4/2
  Product3/1 -> Sum of Elements/1
  Product1/1 -> Sum of Elements/2
  Product2/1 -> Sum of Elements/3
  Product4/1 -> Sum of Elements/4
  Subtract4/1 -> Product3/2, Product3/1
  Subtract5/1 -> Product1/2, Product1/1
  Subtract6/1 -> Product2/2, Product2/1
  Subtract7/1 -> Product4/2, Product4/1

== system cost_function_only/HDL_DUT/Subsystem/Subsystem4 ==
  Prediction_5 : Inport
  id_ref : Inport  Port=2
  iq_ref : Inport  Port=3
  ix_ref : Inport  Port=4
  iy_ref : Inport  Port=5
  Demux : Demux
  Product{1..4} (4 alike) : Product  OutDataTypeStr=fixdt(1,20,11)
  Subtract{4..7} (4 alike) : Sum  Inputs=+-  OutDataTypeStr=fixdt(1,20,11)
  Sum of Elements : Sum  Inputs=++++  OutDataTypeStr=fixdt(1,20,11)
  J5 : Outport
  wires:
  Prediction_5/1 -> Demux/1
  iy_ref/1 -> Subtract7/1
  Demux/3 -> Subtract6/2
  Sum of Elements/1 -> J5/1  "J"
  iq_ref/1 -> Subtract5/1
  id_ref/1 -> Subtract4/1
  Demux/2 -> Subtract5/2
  ix_ref/1 -> Subtract6/1
  Demux/4 -> Subtract7/2
  Demux/1 -> Subtract4/2
  Product3/1 -> Sum of Elements/1
  Product1/1 -> Sum of Elements/2
  Product2/1 -> Sum of Elements/3
  Product4/1 -> Sum of Elements/4
  Subtract4/1 -> Product3/1, Product3/2
  Subtract5/1 -> Product1/2, Product1/1
  Subtract6/1 -> Product2/2, Product2/1
  Subtract7/1 -> Product4/2, Product4/1

== system cost_function_only/HDL_DUT/Subsystem/Subsystem5 ==
  Prediction_6 : Inport
  id_ref : Inport  Port=2
  iq_ref : Inport  Port=3
  ix_ref : Inport  Port=4
  iy_ref : Inport  Port=5
  Demux : Demux
  Product{1..4} (4 alike) : Product  OutDataTypeStr=fixdt(1,20,11)
  Subtract{4..7} (4 alike) : Sum  Inputs=+-  OutDataTypeStr=fixdt(1,20,11)
  Sum of Elements : Sum  Inputs=++++  OutDataTypeStr=fixdt(1,20,11)
  J6 : Outport
  wires:
  Prediction_6/1 -> Demux/1
  iy_ref/1 -> Subtract7/1
  Demux/3 -> Subtract6/2
  Sum of Elements/1 -> J6/1  "J"
  iq_ref/1 -> Subtract5/1
  id_ref/1 -> Subtract4/1
  Demux/2 -> Subtract5/2
  ix_ref/1 -> Subtract6/1
  Demux/4 -> Subtract7/2
  Demux/1 -> Subtract4/2
  Product3/1 -> Sum of Elements/1
  Product1/1 -> Sum of Elements/2
  Product2/1 -> Sum of Elements/3
  Product4/1 -> Sum of Elements/4
  Subtract4/1 -> Product3/2, Product3/1
  Subtract5/1 -> Product1/1, Product1/2
  Subtract6/1 -> Product2/2, Product2/1
  Subtract7/1 -> Product4/2, Product4/1

== system cost_function_only/HDL_DUT/Subsystem/Subsystem6 ==
  Prediction_7 : Inport
  id_ref : Inport  Port=2
  iq_ref : Inport  Port=3
  ix_ref : Inport  Port=4
  iy_ref : Inport  Port=5
  Demux : Demux
  Product{1..4} (4 alike) : Product  OutDataTypeStr=fixdt(1,20,11)
  Subtract{4..7} (4 alike) : Sum  Inputs=+-  OutDataTypeStr=fixdt(1,20,11)
  Sum of Elements : Sum  Inputs=++++  OutDataTypeStr=fixdt(1,20,11)
  J7 : Outport
  wires:
  Prediction_7/1 -> Demux/1
  iy_ref/1 -> Subtract7/1
  Demux/3 -> Subtract6/2
  Sum of Elements/1 -> J7/1  "J"
  iq_ref/1 -> Subtract5/1
  id_ref/1 -> Subtract4/1
  Demux/2 -> Subtract5/2
  ix_ref/1 -> Subtract6/1
  Demux/4 -> Subtract7/2
  Demux/1 -> Subtract4/2
  Product3/1 -> Sum of Elements/1
  Product1/1 -> Sum of Elements/2
  Product2/1 -> Sum of Elements/3
  Product4/1 -> Sum of Elements/4
  Subtract4/1 -> Product3/2, Product3/1
  Subtract5/1 -> Product1/2, Product1/1
  Subtract6/1 -> Product2/2, Product2/1
  Subtract7/1 -> Product4/2, Product4/1

== system cost_function_only/HDL_DUT/Subsystem/Subsystem7 ==
  Prediction_8 : Inport
  id_ref : Inport  Port=2
  iq_ref : Inport  Port=3
  ix_ref : Inport  Port=4
  iy_ref : Inport  Port=5
  Demux : Demux
  Product{1..4} (4 alike) : Product  OutDataTypeStr=fixdt(1,20,11)
  Subtract{4..7} (4 alike) : Sum  Inputs=+-  OutDataTypeStr=fixdt(1,20,11)
  Sum of Elements : Sum  Inputs=++++  OutDataTypeStr=fixdt(1,20,11)
  J8 : Outport
  wires:
  Prediction_8/1 -> Demux/1
  iy_ref/1 -> Subtract7/1
  Demux/3 -> Subtract6/2
  Sum of Elements/1 -> J8/1  "J"
  iq_ref/1 -> Subtract5/1
  id_ref/1 -> Subtract4/1
  Demux/2 -> Subtract5/2
  ix_ref/1 -> Subtract6/1
  Demux/4 -> Subtract7/2
  Demux/1 -> Subtract4/2
  Product3/1 -> Sum of Elements/1
  Product1/1 -> Sum of Elements/2
  Product2/1 -> Sum of Elements/3
  Product4/1 -> Sum of Elements/4
  Subtract4/1 -> Product3/1, Product3/2
  Subtract5/1 -> Product1/1, Product1/2
  Subtract6/1 -> Product2/1, Product2/2
  Subtract7/1 -> Product4/2, Product4/1

== system cost_function_only/HDL_DUT/Subsystem/Subsystem8 ==
  Prediction_9 : Inport
  id_ref : Inport  Port=2
  iq_ref : Inport  Port=3
  ix_ref : Inport  Port=4
  iy_ref : Inport  Port=5
  Demux : Demux
  Product{1..4} (4 alike) : Product  OutDataTypeStr=fixdt(1,20,11)
  Subtract{4..7} (4 alike) : Sum  Inputs=+-  OutDataTypeStr=fixdt(1,20,11)
  Sum of Elements : Sum  Inputs=++++  OutDataTypeStr=fixdt(1,20,11)
  J9 : Outport
  wires:
  Prediction_9/1 -> Demux/1
  iy_ref/1 -> Subtract7/1
  Demux/3 -> Subtract6/2
  Sum of Elements/1 -> J9/1  "J"
  iq_ref/1 -> Subtract5/1
  id_ref/1 -> Subtract4/1
  Demux/2 -> Subtract5/2
  ix_ref/1 -> Subtract6/1
  Demux/4 -> Subtract7/2
  Demux/1 -> Subtract4/2
  Product3/1 -> Sum of Elements/1
  Product1/1 -> Sum of Elements/2
  Product2/1 -> Sum of Elements/3
  Product4/1 -> Sum of Elements/4
  Subtract4/1 -> Product3/2, Product3/1
  Subtract5/1 -> Product1/2, Product1/1
  Subtract6/1 -> Product2/2, Product2/1
  Subtract7/1 -> Product4/2, Product4/1

== system cost_function_only/HDL_DUT/Subsystem/Subsystem9 ==
  Prediction_10 : Inport
  id_ref : Inport  Port=2
  iq_ref : Inport  Port=3
  ix_ref : Inport  Port=4
  iy_ref : Inport  Port=5
  Demux : Demux
  Product{1..4} (4 alike) : Product  OutDataTypeStr=fixdt(1,20,11)
  Subtract{4..7} (4 alike) : Sum  Inputs=+-  OutDataTypeStr=fixdt(1,20,11)
  Sum of Elements : Sum  Inputs=++++  OutDataTypeStr=fixdt(1,20,11)
  J10 : Outport
  wires:
  Prediction_10/1 -> Demux/1
  iy_ref/1 -> Subtract7/1
  Demux/3 -> Subtract6/2
  Sum of Elements/1 -> J10/1  "J"
  iq_ref/1 -> Subtract5/1
  id_ref/1 -> Subtract4/1
  Demux/2 -> Subtract5/2
  ix_ref/1 -> Subtract6/1
  Demux/4 -> Subtract7/2
  Demux/1 -> Subtract4/2
  Product3/1 -> Sum of Elements/1
  Product1/1 -> Sum of Elements/2
  Product2/1 -> Sum of Elements/3
  Product4/1 -> Sum of Elements/4
  Subtract4/1 -> Product3/2, Product3/1
  Subtract5/1 -> Product1/2, Product1/1
  Subtract6/1 -> Product2/2, Product2/1
  Subtract7/1 -> Product4/2, Product4/1
